simulink model "Comfort-oriented_Cruise_Control_Sim"  (R2018b)
settings: Solver=VariableStepAuto  StartTime=0.0  StopTime=2500  RelTol=1e-3
values from neighbouring files (symbols this model uses):
  a1 = 2*pi*n_c    (= 0.0628318530718)    [Comfort-orientedCruise_Control.m]
  Area = 2.4    [Comfort-orientedCruise_Control.m]
  Aver = [0 1 0 0; [-k -c k c]/ms; 0 0 0 1; [k c -k-kt -c]/mus]    [Comfort-orientedCruise_Control.m]
  b1 = 2*pi*n_0*sqrt(Gd)    [Comfort-orientedCruise_Control.m]
  Bver = [0 0; [0 -actuator]/ms; 0 0; [kt actuator]/mus]    [Comfort-orientedCruise_Control.m]
  CrN = 0.01    [Comfort-orientedCruise_Control.m]
  Cv = 0.32    [Comfort-orientedCruise_Control.m]    (also in main.m)
  Cver = [Aver(2,:); 0 1 0 0; 1 0 0 0; 0 0 0 1; 0 0 1 0; 0 1 0 -1; 1 0 -1 0]    [Comfort-orientedCruise_Control.m]
  delayN = 0.2    [Comfort-orientedCruise_Control.m]
  Dver = [Bver(2,:); 0 0 ; 0 0; 0 0; 0 0; 0 0; 0 0]    [Comfort-orientedCruise_Control.m]
  F = zeros(length(mGrid), length(v0Grid))    [Comfort-orientedCruise_Control.m]
  FMax = 4000    [Comfort-orientedCruise_Control.m]    (also in main.m = 5000)
  g = 9.81    [Comfort-orientedCruise_Control.m]    (also in main.m)
  H = zeros(length(mGrid), length(v0Grid))    [Comfort-orientedCruise_Control.m]
  mGrid = m    [Comfort-orientedCruise_Control.m]
  mi = 1480    [Comfort-orientedCruise_Control.m]
  rho = 1.3    [Comfort-orientedCruise_Control.m]
  tauActN = 0.1    [Comfort-orientedCruise_Control.m]
  updateDistance = 1000    [Comfort-orientedCruise_Control.m]
  v0Grid = 0 : 3 : 30    [Comfort-orientedCruise_Control.m]
  windAveN = 12/3.6    (= 3.33333333333)    [Comfort-orientedCruise_Control.m]
libraries: simulink x4, cstblocks x1
settings Model: Creator=senameo  LastModifiedBy=senameo

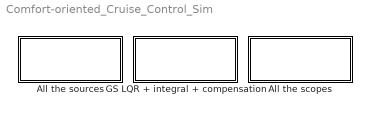
== system Comfort-oriented_Cruise_Control_Sim ==
  All the scopes : Subsystem
  All the sources : Subsystem
  GS LQR + integral + compensation : Subsystem

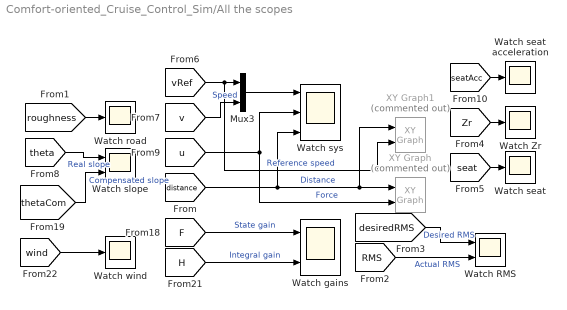
== system Comfort-oriented_Cruise_Control_Sim/All the scopes ==
  Mux3 : Mux  Inputs=2
  Watch RMS : Scope  NumInputPorts=2
  Watch Zr : Scope
  Watch gains : Scope  NumInputPorts=2
  Watch road : Scope
  Watch seat : Scope
  Watch seat acceleration : Scope
  Watch slope : Scope  NumInputPorts=2
  Watch sys : Scope  NumInputPorts=3
  Watch wind : Scope
  XY Graph : simulink/Sinks/XY Graph  Commented=on  xmin=-inf  xmax=inf  ymin=-inf  ymax=inf  st=-1
  XY Graph1 : simulink/Sinks/XY Graph  Commented=on  xmin=-inf  xmax=inf  ymin=-inf  ymax=inf  st=-1
  wires:
  [vRef] -> XY Graph1/2, Mux3/1  "Reference speed"
  Mux3/1 -> Watch sys/1
  [v] -> Mux3/2  "Speed"
  [u] -> XY Graph/2, Watch sys/2  "Force"
  [F] -> Watch gains/1  "State gain"
  [H] -> Watch gains/2  "Integral gain"
  [theta] -> Watch slope/1  "Real slope"
  [thetaCom] -> Watch slope/2  "Compensated slope"
  [wind] -> Watch wind/1
  [roughness] -> Watch road/1
  [distance] -> Watch sys/3, XY Graph1/1, XY Graph/1  "Distance"
  [RMS] -> Watch RMS/2  "Actual RMS"
  [desiredRMS] -> Watch RMS/1  "Desired RMS"
  [Zr] -> Watch Zr/1
  [seat] -> Watch seat/1
  [seatAcc] -> Watch seat acceleration/1

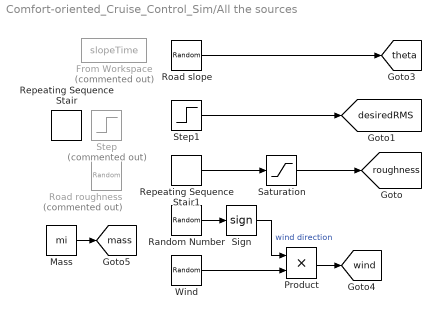
== system Comfort-oriented_Cruise_Control_Sim/All the sources ==
  From Workspace : FromWorkspace  Commented=on  VariableName=slopeTime  SampleTime=0
  Mass : Constant  Value=mi
  Product : Product
  Random Number : RandomNumber  Variance=0.1  SampleTime=1
  Repeating Sequence Stair : simulink/Sources/Repeating Sequence Stair  OutValues=[0.3 0.6 0.9].'  tsamp=720  OutMin=[]  OutMax=[]  OutDataTypeStr=double  OutputDataTypeScalingMode=double  OutDataType=fixdt(0,8)  ConRadixGroup=Best Precision: Vector-wise  OutScaling=2^-12
  Repeating Sequence Stair1 : simulink/Sources/Repeating Sequence Stair  OutValues=1e-6*[10 20 50 200]  tsamp=360  OutMin=[]  OutMax=[]  OutDataTypeStr=double  OutputDataTypeScalingMode=double  OutDataType=fixdt(0,8)  ConRadixGroup=Best Precision: Vector-wise  OutScaling=2^-12
  Road roughness : RandomNumber  Commented=on  Variance=0.0000001/10
  Road slope : RandomNumber  Variance=0.002  SampleTime=1
  Saturation : Saturate  UpperLimit=1617e-6  LowerLimit=0
  Sign : Signum
  Step : Step  Commented=on  Time=250  Before=0.315  After=0.8  SampleTime=0
  Step1 : Step  Time=1000  Before=0.6  After=0.3  SampleTime=0
  Wind : RandomNumber  Mean=windAveN  Variance=10  SampleTime=1
  tag scope: desiredRMS=global, mass=global, roughness=global, theta=global, wind=global
  wires:
  Mass/1 -> [mass]
  Random Number/1 -> Sign/1
  Wind/1 -> Product/2
  Sign/1 -> Product/1  "wind direction"
  Product/1 -> [wind]
  Road slope/1 -> [theta]
  Repeating Sequence Stair1/1 -> Saturation/1
  Step1/1 -> [desiredRMS]
  Saturation/1 -> [roughness]

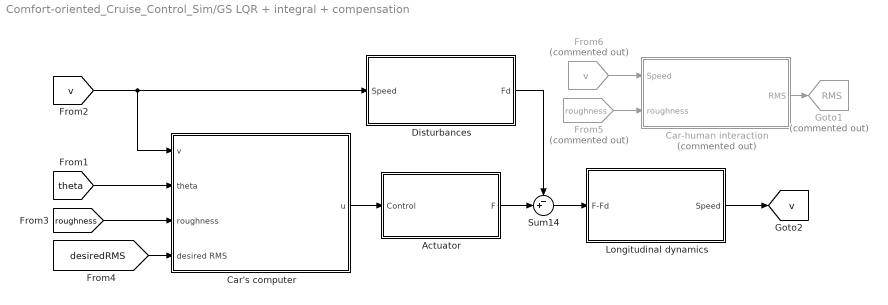
== system Comfort-oriented_Cruise_Control_Sim/GS LQR + integral + compensation ==
  Actuator : Subsystem
  Car's computer : Subsystem
  Car-human interaction : Subsystem  Commented=on
  Disturbances : Subsystem
  From5 : From  Commented=on  GotoTag=roughness  TagVisibility=global
  From6 : From  Commented=on  GotoTag=v  TagVisibility=global
  Goto1 : Goto  Commented=on  GotoTag=RMS  TagVisibility=global
  Longitudinal dynamics : Subsystem
  Sum14 : Sum  Inputs=-+|
  tag scope: v=global
  wires:
  Disturbances/1(Fd) -> Sum14/1
  [v] -> Car's computer/1(v), Disturbances/1(Speed)
  Actuator/1(F) -> Sum14/2
  Sum14/1 -> Longitudinal dynamics/1("F-Fd ")
  Longitudinal dynamics/1(Speed) -> [v]
  Car's computer/1(u) -> Actuator/1(Control)
  [theta] -> Car's computer/2(theta)
  [roughness] -> Car's computer/3(roughness)
  [desiredRMS] -> Car's computer/4(desired RMS)
  From5/1 -> Car-human interaction/2(roughness)
  From6/1 -> Car-human interaction/1(Speed)
  Car-human interaction/1(RMS) -> Goto1/1

== system Comfort-oriented_Cruise_Control_Sim/GS LQR + integral + compensation/Actuator ==
  Control : Inport
  Actuator : TransferFcn  Denominator=[tauActN 1]
  Saturation : Saturate  UpperLimit=FMax  LowerLimit=-FMax
  Transport Delay1 : TransportDelay  DelayTime=delayN
  F : Outport
  tag scope: u=global
  wires:
  Control/1 -> Actuator/1
  Saturation/1 -> Transport Delay1/1
  Actuator/1 -> Saturation/1  "F"
  Transport Delay1/1 -> [u], F/1

== system Comfort-oriented_Cruise_Control_Sim/GS LQR + integral + compensation/Car's computer ==
  v : Inport
  theta : Inport  Port=2
  roughness : Inport  Port=3
  desired RMS : Inport  Port=4
  Comfort-based reference speed calculator : Subsystem
  Distance tracker : Subsystem
  Longitudinal controller : Subsystem
  u : Outport
  wires:
  Longitudinal controller/1(u) -> u/1
  ? -> Longitudinal controller/2(vRef)
  v/1 -> Longitudinal controller/1(v), Distance tracker/1(v)
  roughness/1 -> Comfort-based reference speed calculator/1(roughness)
  theta/1 -> Longitudinal controller/3(theta)
  desired RMS/1 -> Comfort-based reference speed calculator/2(desired RMS)

== system Comfort-oriented_Cruise_Control_Sim/GS LQR + integral + compensation/Car-human interaction ==
  Speed : Inport
  roughness : Inport  Port=2
  Human body : Subsystem
  Road to Car (space domain equations) : Subsystem
  Vertical dynamics : Subsystem
  Vertical suspension : Subsystem
  RMS : Outport  VectorParamsAs1DForOutWhenUnconnected=on
  wires:
  Speed/1 -> Road to Car (space domain equations)/1(Speed)
  roughness/1 -> Road to Car (space domain equations)/2(roughness)
  Road to Car (space domain equations)/1(Zr) -> Vertical dynamics/1(Zr)
  Vertical dynamics/1(a) -> Human body/1(a)
  Vertical suspension/1(uV) -> Vertical dynamics/2(uV)
  Human body/1(RMS acceleration) -> RMS/1

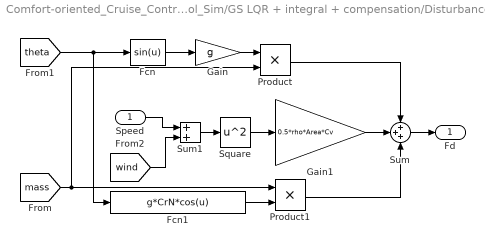
== system Comfort-oriented_Cruise_Control_Sim/GS LQR + integral + compensation/Disturbances ==
  Speed : Inport
  Fcn : Fcn  Expr=sin(u)
  Fcn1 : Fcn  Expr=g*CrN*cos(u)
  Gain : Gain  Gain=g
  Gain1 : Gain  Gain=0.5*rho*Area*Cv
  Product : Product
  Product1 : Product
  Square : Math  Operator=square  SaturateOnIntegerOverflow=on
  Sum : Sum  Inputs=+++
  Sum1 : Sum
  Fd : Outport
  wires:
  [wind] -> Sum1/2
  Product1/1 -> Sum/3
  Fcn1/1 -> Product1/2
  [mass] -> Product/2, Product1/1
  Gain/1 -> Product/1
  Product/1 -> Sum/1
  Speed/1 -> Sum1/1
  Sum1/1 -> Square/1
  Fcn/1 -> Gain/1
  Sum/1 -> Fd/1
  Gain1/1 -> Sum/2
  Square/1 -> Gain1/1
  [theta] -> Fcn/1, Fcn1/1

== system Comfort-oriented_Cruise_Control_Sim/GS LQR + integral + compensation/Longitudinal dynamics ==
  "F-Fd " : Inport
  Divide : Product  Inputs=*/
  Integrator1 : Integrator  InitialCondition=25
  Speed : Outport
  tag scope: ac_longi=global
  wires:
  Divide/1 -> [ac_longi], Integrator1/1  "v dot"
  "F-Fd "/1 -> Divide/1  "F-Fd"
  Integrator1/1 -> Speed/1  "Speed"
  [mass] -> Divide/2

== system Comfort-oriented_Cruise_Control_Sim/GS LQR + integral + compensation/Car's computer/Comfort-based reference speed calculator ==
  roughness : Inport
  desired RMS : Inport  Port=2
  Demux : Demux  Outputs=3
  MATLAB Function : MATLAB Function  TreatAsAtomicUnit=on
  Mux : Mux  Inputs=2
  vref : Outport
  wires:
  Mux/1 -> MATLAB Function/1(u)
  MATLAB Function/1(y) -> Demux/1
  Demux/2 -> ?
  Demux/3 -> ?
  Demux/1 -> vref/1
  roughness/1 -> Mux/1  "Road  geometric  mean"
  desired RMS/1 -> Mux/2

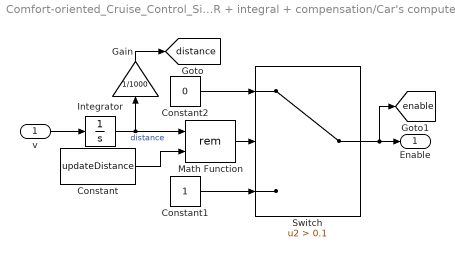
== system Comfort-oriented_Cruise_Control_Sim/GS LQR + integral + compensation/Car's computer/Distance tracker ==
  v : Inport
  Constant : Constant  Value=updateDistance
  Constant1 : Constant
  Constant2 : Constant  Value=0
  Gain : Gain  Gain=1/1000
  Integrator : Integrator
  Math Function : Math  Operator=rem  OutputSignalType=real  SaturateOnIntegerOverflow=on
  Switch : Switch  Criteria=u2 > Threshold  Threshold=0.1
  Enable : Outport  VectorParamsAs1DForOutWhenUnconnected=on
  tag scope: distance=global, enable=global
  wires:
  Constant/1 -> Math Function/2
  Math Function/1 -> Switch/2
  v/1 -> Integrator/1
  Integrator/1 -> Gain/1, Math Function/1  "distance"
  Switch/1 -> [enable], Enable/1
  Constant2/1 -> Switch/1
  Constant1/1 -> Switch/3
  Gain/1 -> [distance]

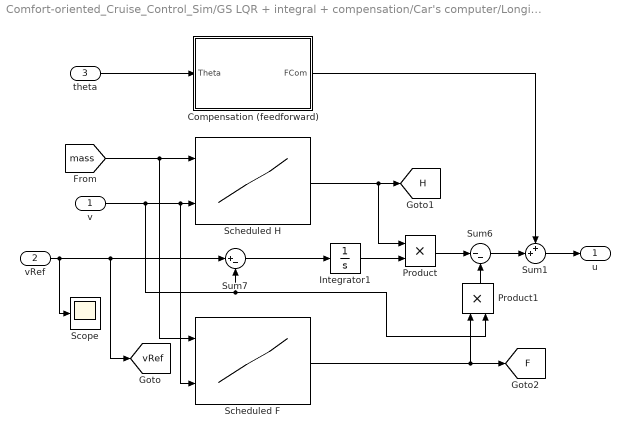
== system Comfort-oriented_Cruise_Control_Sim/GS LQR + integral + compensation/Car's computer/Longitudinal controller ==
  v : Inport
  vRef : Inport  Port=2
  theta : Inport  Port=3
  "Compensation (feedforward) " : Subsystem
  Integrator1 : Integrator
  Product : Product
  Product1 : Product
  Scheduled F : Lookup_n-D  BreakpointsForDimension1=mGrid  BreakpointsForDimension2=v0Grid  Table=F  InternalRulePriority=Speed  RndMeth=Simplest  InputSameDT=on
  Scheduled H : Lookup_n-D  BreakpointsForDimension1=mGrid  BreakpointsForDimension2=v0Grid  Table=H  InternalRulePriority=Speed  RndMeth=Simplest  InputSameDT=on
  Scope : Scope
  Sum1 : Sum  Inputs=++|
  Sum6 : Sum  Inputs=|--
  Sum7 : Sum  Inputs=|+-
  u : Outport
  tag scope: F=global, H=global, vRef=global
  wires:
  Scheduled H/1 -> Product/1, [H]
  v/1 -> Scheduled F/2, Scheduled H/2, Sum7/2, Product1/2
  [mass] -> Scheduled H/1, Scheduled F/1
  Product1/1 -> Sum6/2
  Product/1 -> Sum6/1
  Scheduled F/1 -> [F], Product1/1
  Integrator1/1 -> Product/2
  "Compensation (feedforward) "/1(FCom) -> Sum1/1
  Sum6/1 -> Sum1/2
  Sum1/1 -> u/1
  Sum7/1 -> Integrator1/1
  theta/1 -> "Compensation (feedforward) "/1(Theta)
  vRef/1 -> Scope/1, [vRef], Sum7/1

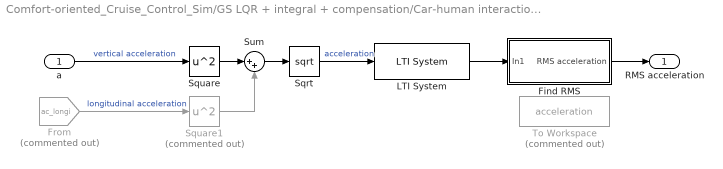
== system Comfort-oriented_Cruise_Control_Sim/GS LQR + integral + compensation/Car-human interaction/Human body ==
  a : Inport
  Find RMS : Subsystem
  From : From  Commented=on  GotoTag=ac_longi  TagVisibility=global
  LTI System : cstblocks/LTI System  sys=WISO_2631  IC=[]
  Sqrt : Sqrt  SaturateOnIntegerOverflow=on
  Square : Math  Operator=square  SaturateOnIntegerOverflow=on
  Square1 : Math  Commented=on  Operator=square  SaturateOnIntegerOverflow=on
  Sum : Sum  Inputs=|++
  To Workspace : ToWorkspace  Commented=on  VariableName=acceleration  SaveFormat=Structure With Time  SampleTime=-1
  RMS acceleration : Outport  VectorParamsAs1DForOutWhenUnconnected=on
  wires:
  a/1 -> Square/1  "vertical acceleration"
  From/1 -> Square1/1  "longitudinal acceleration"
  Sum/1 -> Sqrt/1
  Sqrt/1 -> LTI System/1  "acceleration"
  LTI System/1 -> Find RMS/1(In1)
  Square/1 -> Sum/1
  Find RMS/1(RMS acceleration) -> RMS acceleration/1
  Square1/1 -> Sum/2

== system Comfort-oriented_Cruise_Control_Sim/GS LQR + integral + compensation/Car-human interaction/Road to Car (space domain equations) ==
  Speed : Inport
  roughness : Inport  Port=2
  "\tISO road profile classification" : If  IfExpression=0 < u1 <= 25.3e-6  ElseIfExpressions=25.3e-6 < u1 <= 101.1e-6, 101.1e-6 < u1 <= 404.3e-6
  " Class AB" : Subsystem  TreatAsAtomicUnit=on
  Class C : Subsystem  TreatAsAtomicUnit=on
  Class D : Subsystem  TreatAsAtomicUnit=on
  Class E : Subsystem  TreatAsAtomicUnit=on
  Sum : Sum  Inputs=++++
  Zr : Outport
  wires:
  "\tISO road profile classification"/2 -> Class C/Action
  " Class AB"/1(Zr if AB) -> Sum/1
  roughness/1 -> "\tISO road profile classification"/1  "Road  geometric  mean"
  Class D/1(Zr if D) -> Sum/3
  "\tISO road profile classification"/3 -> Class D/Action
  "\tISO road profile classification"/4 -> Class E/Action
  Class E/1(Zr if E) -> Sum/4
  Sum/1 -> Zr/1
  "\tISO road profile classification"/1 -> " Class AB"/Action
  Class C/1(Zr if C) -> Sum/2
  Speed/1 -> Class E/1(speed), Class D/1(speed), " Class AB"/1(speed), Class C/1(speed)

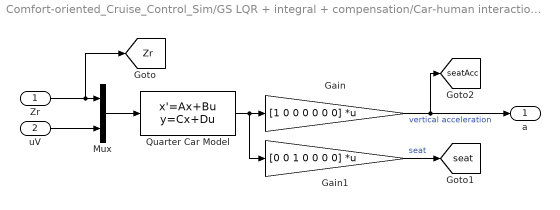
== system Comfort-oriented_Cruise_Control_Sim/GS LQR + integral + compensation/Car-human interaction/Vertical dynamics ==
  Zr : Inport
  uV : Inport  Port=2
  Gain : Gain  Gain=[1 0 0 0 0 0 0]  Multiplication=Matrix(K*u) (u vector)
  Gain1 : Gain  Gain=[0 0 1 0 0 0 0]  Multiplication=Matrix(K*u) (u vector)
  Mux : Mux  Inputs=2
  Quarter Car Model : StateSpace  A=Aver  B=Bver  C=Cver  D=Dver  InitialCondition=0
  a : Outport  VectorParamsAs1DForOutWhenUnconnected=on
  tag scope: Zr=global, seat=global, seatAcc=global
  wires:
  Zr/1 -> [Zr], Mux/1
  Mux/1 -> Quarter Car Model/1
  uV/1 -> Mux/2
  Gain/1 -> [seatAcc], a/1  "vertical acceleration"
  Quarter Car Model/1 -> Gain1/1, Gain/1
  Gain1/1 -> [seat]  "seat"

== system Comfort-oriented_Cruise_Control_Sim/GS LQR + integral + compensation/Car-human interaction/Vertical suspension ==
  u_vertical : Step  Time=0  After=0  SampleTime=0
  uV : Outport  VectorParamsAs1DForOutWhenUnconnected=on
  wires:
  u_vertical/1 -> uV/1  "vertical control"

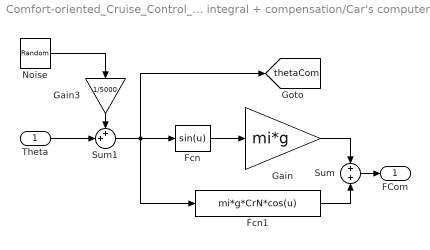
== system Comfort-oriented_Cruise_Control_Sim/GS LQR + integral + compensation/Car's computer/Longitudinal controller/Compensation (feedforward)  ==
  Theta : Inport
  Fcn : Fcn  Expr=sin(u)
  Fcn1 : Fcn  Expr=mi*g*CrN*cos(u)
  Gain : Gain  Gain=mi*g
  Gain3 : Gain  Gain=1/5000
  Noise : RandomNumber  Variance=10  SampleTime=0.1
  Sum : Sum  Inputs=+|+
  Sum1 : Sum  Inputs=++|
  FCom : Outport
  tag scope: thetaCom=global
  wires:
  Gain/1 -> Sum/1
  Fcn1/1 -> Sum/2
  Fcn/1 -> Gain/1
  Sum/1 -> FCom/1
  Noise/1 -> Gain3/1
  Gain3/1 -> Sum1/1
  Theta/1 -> Sum1/2
  Sum1/1 -> [thetaCom], Fcn1/1, Fcn/1

== system Comfort-oriented_Cruise_Control_Sim/GS LQR + integral + compensation/Car-human interaction/Human body/Find RMS ==
  In1 : Inport
  Constant : Constant
  Divide : Product  Inputs=*/
  Integrator : Integrator  ExternalReset=rising
  Integrator1 : Integrator  ExternalReset=rising
  Square : Math  Operator=square  SaturateOnIntegerOverflow=on
  Square Root : Sqrt  SaturateOnIntegerOverflow=on
  RMS acceleration : Outport  VectorParamsAs1DForOutWhenUnconnected=on
  wires:
  Square/1 -> Integrator/1
  Integrator/1 -> Divide/1
  Divide/1 -> Square Root/1
  In1/1 -> Square/1
  [enable] -> Integrator1/2, Integrator/2
  Constant/1 -> Integrator1/1
  Integrator1/1 -> Divide/2  "Reset period"
  Square Root/1 -> RMS acceleration/1

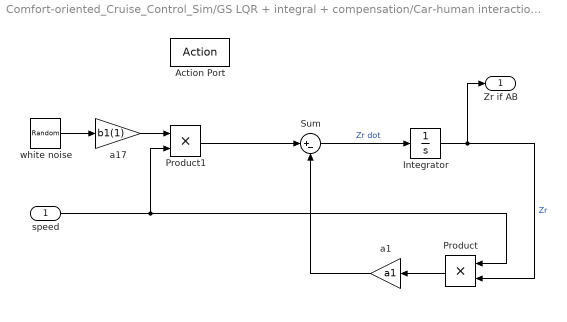
== system Comfort-oriented_Cruise_Control_Sim/GS LQR + integral + compensation/Car-human interaction/Road to Car (space domain equations)/ Class AB ==
  speed : Inport
  Action Port : ActionPort
  Integrator : Integrator
  Product : Product
  Product1 : Product
  Sum : Sum  Inputs=|+-
  a1 : Gain  Gain=a1
  a17 : Gain  Gain=b1(1)
  "white noise " : RandomNumber
  Zr if AB : Outport  VectorParamsAs1DForOutWhenUnconnected=on
  wires:
  "white noise "/1 -> a17/1
  a1/1 -> Sum/2
  Sum/1 -> Integrator/1  "Zr dot"
  Product1/1 -> Sum/1
  Integrator/1 -> Zr if AB/1, Product/2  "Zr"
  Product/1 -> a1/1
  a17/1 -> Product1/1
  speed/1 -> Product/1, Product1/2

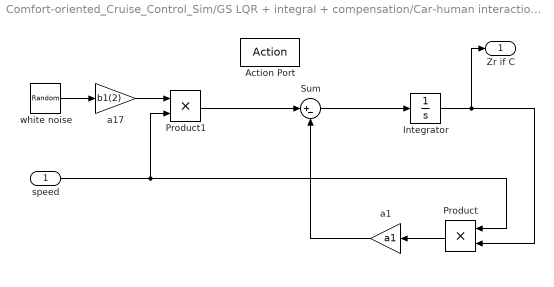
== system Comfort-oriented_Cruise_Control_Sim/GS LQR + integral + compensation/Car-human interaction/Road to Car (space domain equations)/Class C ==
  speed : Inport
  Action Port : ActionPort
  Integrator : Integrator
  Product : Product
  Product1 : Product
  Sum : Sum  Inputs=|+-
  a1 : Gain  Gain=a1
  a17 : Gain  Gain=b1(2)
  "white noise " : RandomNumber
  Zr if C : Outport  VectorParamsAs1DForOutWhenUnconnected=on
  wires:
  Product/1 -> a1/1
  "white noise "/1 -> a17/1
  Sum/1 -> Integrator/1
  a1/1 -> Sum/2
  Integrator/1 -> Zr if C/1, Product/2
  Product1/1 -> Sum/1
  a17/1 -> Product1/1
  speed/1 -> Product/1, Product1/2

== system Comfort-oriented_Cruise_Control_Sim/GS LQR + integral + compensation/Car-human interaction/Road to Car (space domain equations)/Class D ==
  speed : Inport
  Action Port : ActionPort
  Integrator : Integrator
  Product : Product
  Product1 : Product
  Sum : Sum  Inputs=|+-
  a1 : Gain  Gain=a1
  a17 : Gain  Gain=b1(3)
  "white noise " : RandomNumber
  Zr if D : Outport  VectorParamsAs1DForOutWhenUnconnected=on
  wires:
  Product/1 -> a1/1
  "white noise "/1 -> a17/1
  Sum/1 -> Integrator/1
  a1/1 -> Sum/2
  Integrator/1 -> Zr if D/1, Product/2
  Product1/1 -> Sum/1
  a17/1 -> Product1/1
  speed/1 -> Product/1, Product1/2

== system Comfort-oriented_Cruise_Control_Sim/GS LQR + integral + compensation/Car-human interaction/Road to Car (space domain equations)/Class E ==
  speed : Inport
  Action Port : ActionPort
  Integrator : Integrator
  Product : Product
  Product1 : Product
  Sum : Sum  Inputs=|+-
  a1 : Gain  Gain=a1
  a17 : Gain  Gain=b1(4)
  "white noise " : RandomNumber
  Zr if E : Outport  VectorParamsAs1DForOutWhenUnconnected=on
  wires:
  Product/1 -> a1/1
  "white noise "/1 -> a17/1
  Sum/1 -> Integrator/1
  a1/1 -> Sum/2
  Integrator/1 -> Zr if E/1, Product/2
  Product1/1 -> Sum/1
  a17/1 -> Product1/1
  speed/1 -> Product/1, Product1/2

== matlab function Comfort-oriented_Cruise_Control_Sim/GS LQR + integral + compensation/Car's computer/Comfort-based reference speed calculator/MATLAB Function ==
  data: u input; y output
function y = fcn(u)
poli_road_A =[-2.810588227248419e+05,6.169326456562061e+05,-5.532877354090116e+05,2.592697706189919e+05,-6.700633721138796e+04,9.126098470124590e+03,-4.908206795592492e+02,17.034337618461410];
poli_road_B=[-2.918464207163787e+03,1.256660289518003e+04,-2.213392570093140e+04,2.042007729169009e+04,-1.043888402402951e+04,2.839027450728016e+03,-3.194031408439325e+02,20.363551425734784];
poli_road_C=[-20.580699008933195,1.768188289251797e+02,-6.209471832216163e+02,1.140851851658809e+03,-1.158899742214876e+03,6.230583939060465e+02,-1.343821697265132e+02,17.843722322086556];
poli_road_D=[-0.189767159734969,3.220641909579672,-22.334773208111000,81.060950477925270,-1.629224058712685e+02,1.740926522486322e+02,-76.471563472280050,19.565680049932546];
rho=u(1);
comf=u(2);
vref=0;
if (0 <= rho) & (rho <= 12.3e-6)
   vref=polyval(poli_road_A,comf);
elseif (12.3e-6 < rho) & (rho <= 25.3e-6)
    vref=polyval(poli_road_B,comf);
elseif (25.3e-6 < rho) & (rho <= 101.1e-6)
    vref=polyval(poli_road_C,comf);
elseif (101.1e-6 < rho) & (rho <= 404.3e-6)
    vref=polyval(poli_road_D,comf);
end
y=[vref;rho;comf];
